simulink model "ControlRetroEstadosEscalon - copia"  (R2017b)
settings: Solver=ode45  StartTime=0.0  StopTime=10.0  RelTol=1e-3
values from neighbouring files (symbols this model uses):
  A = double(A)    [Linealizacion.m]
  B = double(B)    [Linealizacion.m]
  C = double(C)    [Linealizacion.m]
  K = acker(Agorrito,Bgorrito,roots(PD))    [Linealizacion.m]
  K1 = acker(Agorrito1,Bgorrito1,roots(PD1))    [Linealizacion.m]
  K2 = acker(Agorrito2,Bgorrito2,roots(PD2))    [Linealizacion.m]
  L1 = acker(A',C',roots(PDobs))'    [Linealizacion.m]
settings Model: Creator=Cx001la  LastModifiedBy=Cx001la

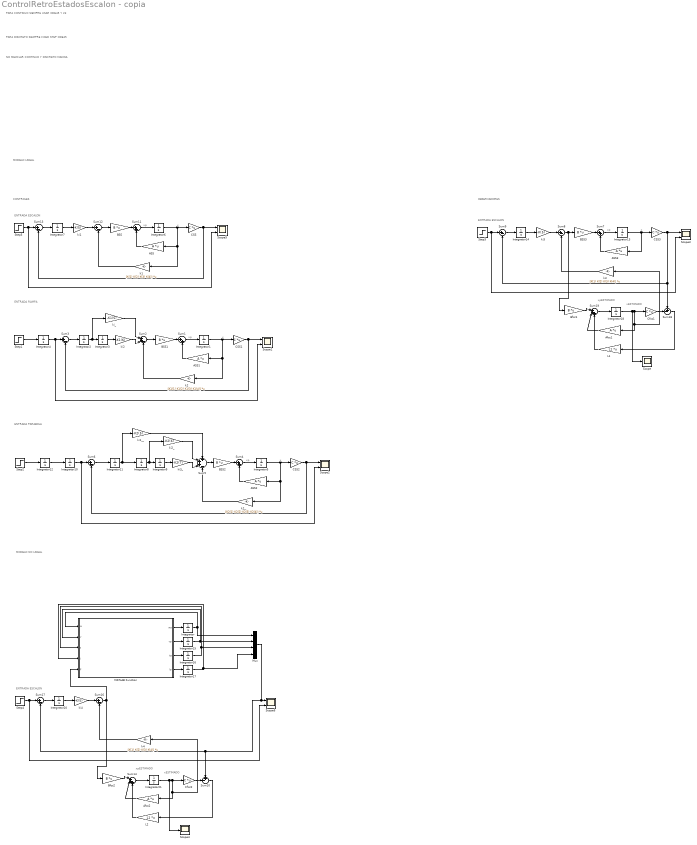
== system ControlRetroEstadosEscalon - copia ==
  note: MODELO LINEAL
  note: PARA DISCRETO SIEMPRE FIXED STEP ODE45
  note: OBSERVADORES
  note: ENTRADA ESCALON
  note: xp
  note: x
  note: ENTRADA RAMPA
  note: x
  note: xp
  note: x
  note: ENTRADA PARABOLA
  note: xp
  note: CONTROLES
  note: ENTRADA ESCALON
  note: x
  note: xp
  note: xpESTIMADO
  note: xESTIMADO
  note: PARA CONTINUO SIEMPRE USAR ODE45 Y 23
  note: NO MEZCLAR CONTINUO Y DISCRETO MAKINA
  note: MODELO NO LINEAL
  note: xESTIMADO
  note: xpESTIMADO
  note: ENTRADA ESCALON
  ASS{,1..3} (4 alike) : Gain  Gain=A  Multiplication=Matrix(K*u)
  Afcc1 : Gain  Gain=A  Multiplication=Matrix(K*u)
  Afcc2 : Gain  Gain=A  Multiplication=Matrix(K*u)
  BSS{,1..3} (4 alike) : Gain  Gain=B  Multiplication=Matrix(K*u)
  Bfcc1 : Gain  Gain=B  Multiplication=Matrix(K*u)
  Bfcc2 : Gain  Gain=B  Multiplication=Matrix(K*u)
  CSS{,1..3} (4 alike) : Gain  Gain=C  Multiplication=Matrix(K*u)
  Cfcc1 : Gain  Gain=C  Multiplication=Matrix(K*u)
  Cfcc2 : Gain  Gain=C  Multiplication=Matrix(K*u)
  Integrator{,1..18,20..21} (21 alike) : Integrator
  L1 : Gain  Gain=L1  Multiplication=Matrix(K*u)
  L2 : Gain  Gain=L1  Multiplication=Matrix(K*u)
  MATLAB Function : MATLAB Function  TreatAsAtomicUnit=on
  Mux : Mux
  Scope : Scope
  Scope{1..3,5..6} (5 alike) : Scope  NumInputPorts=2
  Scope4 : Scope
  Step{1..5} (5 alike) : Step  Time=0  SampleTime=0
  Sum{1,4,7,11} (4 alike) : Sum  Inputs=|++
  Sum10 : Sum  Inputs=+-|
  Sum{3,6,8..9,12..13,16..17} (8 alike) : Sum  Inputs=|+-
  Sum14 : Sum  Inputs=|+++
  Sum18 : Sum  Inputs=+-|
  Sum19 : Sum  Inputs=|+++
  Sum2 : Sum  Inputs=|++-
  Sum5 : Sum  Inputs=+++-
  k1 : Gain  Gain=[K(1) K(2) K(3) K(4)]  Multiplication=Matrix(K*u)
  k2 : Gain  Gain=[K1(1) K1(2) K1(3) K1(4)]  Multiplication=Matrix(K*u)
  k2__ : Gain  Gain=[K2(1) K2(2) K2(3) K2(4)]  Multiplication=Matrix(K*u)
  k3 : Gain  Gain=[K(1) K(2) K(3) K(4)]  Multiplication=Matrix(K*u)
  k4 : Gain  Gain=[K(1) K(2) K(3) K(4)]  Multiplication=Matrix(K*u)
  ki1 : Gain  Gain=-K(5)
  ki1__ : Gain  Gain=-K2(5)
  ki2 : Gain  Gain=-K1(6)
  ki2_ : Gain  Gain=-K2(6)
  ki3 : Gain  Gain=-K(5)
  ki3_ : Gain  Gain=-K2(7)
  ki4 : Gain  Gain=-K(5)
  ki_ : Gain  Gain=-K1(5)
  wires:
  ASS/1 -> Sum11/2
  Sum13/1 -> Integrator7/1
  ki1/1 -> Sum12/1
  Sum12/1 -> BSS/1
  k1/1 -> Sum12/2
  Integrator7/1 -> ki1/1
  BSS/1 -> Sum11/1
  Step5/1 -> Scope5/2, Sum13/1
  Integrator6/1 -> k1/1, ASS/1, CSS/1
  Sum11/1 -> Integrator6/1
  CSS/1 -> Scope5/1, Sum13/2
  Sum1/1 -> Integrator1/1
  CSS1/1 -> Scope1/1, Sum3/2
  BSS1/1 -> Sum1/1
  Sum2/1 -> BSS1/1
  Sum3/1 -> Integrator2/1
  ASS1/1 -> Sum1/2
  Integrator1/1 -> k2/1, ASS1/1, CSS1/1
  Integrator3/1 -> ki2/1
  Integrator2/1 -> ki_/1, Integrator3/1
  k2/1 -> Sum2/3
  ki2/1 -> Sum2/2
  ki_/1 -> Sum2/1
  Integrator4/1 -> Scope1/2, Sum3/1
  Step1/1 -> Integrator4/1
  Integrator9/1 -> ki3_/1
  ASS2/1 -> Sum4/2
  Integrator5/1 -> k2__/1, ASS2/1, CSS2/1
  Sum6/1 -> Integrator11/1
  Sum5/1 -> BSS2/1
  BSS2/1 -> Sum4/1
  CSS2/1 -> Scope2/1, Sum6/2
  Sum4/1 -> Integrator5/1
  Step2/1 -> Integrator12/1
  Integrator10/1 -> Scope2/2, Sum6/1
  Integrator8/1 -> ki2_/1, Integrator9/1
  Integrator11/1 -> ki1__/1, Integrator8/1
  ki1__/1 -> Sum5/1
  k2__/1 -> Sum5/4
  ki3_/1 -> Sum5/3
  ki2_/1 -> Sum5/2
  Integrator12/1 -> Integrator10/1
  Sum7/1 -> Integrator13/1
  Step3/1 -> Scope3/2, Sum9/1
  BSS3/1 -> Sum7/1
  ki3/1 -> Sum8/1
  k3/1 -> Sum8/2
  Integrator14/1 -> ki3/1
  Sum9/1 -> Integrator14/1
  ASS3/1 -> Sum7/2
  Integrator13/1 -> ASS3/1, CSS3/1
  Sum19/1 -> Integrator18/1
  Sum8/1 -> Bfcc1/1, BSS3/1
  CSS3/1 -> Scope3/1, Sum18/1, Sum9/2
  Sum18/1 -> L1/1
  Integrator18/1 -> Scope/1, k3/1, Afcc1/1, Cfcc1/1
  Cfcc1/1 -> Sum18/2
  Afcc1/1 -> Sum19/2
  L1/1 -> Sum19/3
  Bfcc1/1 -> Sum19/1
  MATLAB Function/1(wp) -> Integrator/1
  MATLAB Function/2(vp) -> Integrator15/1
  MATLAB Function/3(tp) -> Integrator16/1
  MATLAB Function/4(lp) -> Integrator17/1
  Integrator/1 -> Mux/1, MATLAB Function/1(w)
  Integrator15/1 -> Mux/2, MATLAB Function/2(v)
  Integrator16/1 -> Mux/3, MATLAB Function/3(t)
  Integrator17/1 -> Mux/4, MATLAB Function/4(l)
  L2/1 -> Sum14/3
  Cfcc2/1 -> Sum10/2
  Integrator21/1 -> Scope4/1, k4/1, Afcc2/1, Cfcc2/1
  Bfcc2/1 -> Sum14/1
  Sum10/1 -> L2/1
  Sum14/1 -> Integrator21/1
  Sum17/1 -> Integrator20/1
  Step4/1 -> Scope6/2, Sum17/1
  k4/1 -> Sum16/2
  Afcc2/1 -> Sum14/2
  Sum16/1 -> MATLAB Function/5(F), Bfcc2/1
  Integrator20/1 -> ki4/1
  Mux/1 -> Sum10/1, Sum17/2, Scope6/1
  ki4/1 -> Sum16/1

== matlab function ControlRetroEstadosEscalon - copia/MATLAB Function ==
  data: w input; wp output; v input; t input; l input; F input; vp output; tp output; lp output
function [wp,vp,tp,lp] = fcn(w,v,t,l,F)
time=0; a=0; wn=0; 
g=9.81; lo=0.5; k=100; m=1;
wp=(1/l)*(  -2*v*w -(a*wn^2*sin(wn*time)-g)*sin(t)  +F*l );
vp=l*w   -(k/m)*(l-lo)   -(  g-a*wn^2*sin(wn*time)  )*cos(t);
tp=w;
lp=v;
